simulink model "test_final_sift"  (R2015a)
settings: Solver=ode45  StartTime=0.0  StopTime=10.0  RelTol=1e-3
InitFcn:
  | %% DSPBuilder Start
  | alt_dspbuilder_update_model(bdroot)
  | %% DSPBuilder End
libraries: allblocks_alteradspbuilder2 x2309
(part 20 of 27)

== system test_final_sift/sift_octave1/get_descriptor/scale_space/Gaussian_scale4/line_buff ==
  dataIn : Inport
  clken : Inport  Port=2
  Delay : allblocks_alteradspbuilder2/Delay  pipeline=1  pipeline_display=1  ClockPhase=1  use_ena=on  use_sclr=off  allowFloatingPointOverride=on  logOutputs=off  logFile=C:\Users\ASUS\Desktop\sift_fpga\Octave_2\tb_test_final_sift\test%5Ffinal%5Fsift_sift%5Foctave1_get%5Fdescriptor_scale%5Fspace_Gaussian%5Fscale4_line%5Fbuff_Delay.fixedpointlog  use_init=off  reset_value=1
  Delay1 : allblocks_alteradspbuilder2/Delay  pipeline=1  pipeline_display=1  ClockPhase=1  use_ena=on  use_sclr=off  allowFloatingPointOverride=on  logOutputs=off  logFile=C:\Users\ASUS\Desktop\sift_fpga\Octave_2\tb_test_final_sift\test%5Ffinal%5Fsift_sift%5Foctave1_get%5Fdescriptor_scale%5Fspace_Gaussian%5Fscale4_line%5Fbuff_Delay1.fixedpointlog  use_init=off  reset_value=1
  Delay10 : allblocks_alteradspbuilder2/Delay  pipeline=1  pipeline_display=1  ClockPhase=1  use_ena=on  use_sclr=off  allowFloatingPointOverride=on  logOutputs=off  logFile=C:\Users\ASUS\Desktop\sift_fpga\Octave_2\tb_test_final_sift\test%5Ffinal%5Fsift_sift%5Foctave1_get%5Fdescriptor_scale%5Fspace_Gaussian%5Fscale4_line%5Fbuff_Delay10.fixedpointlog  use_init=off  reset_value=1
  Delay11 : allblocks_alteradspbuilder2/Delay  pipeline=1  pipeline_display=1  ClockPhase=1  use_ena=on  use_sclr=off  allowFloatingPointOverride=on  logOutputs=off  logFile=C:\Users\ASUS\Desktop\sift_fpga\Octave_2\tb_test_final_sift\test%5Ffinal%5Fsift_sift%5Foctave1_get%5Fdescriptor_scale%5Fspace_Gaussian%5Fscale4_line%5Fbuff_Delay11.fixedpointlog  use_init=off  reset_value=1
  Delay12 : allblocks_alteradspbuilder2/Delay  pipeline=1  pipeline_display=1  ClockPhase=1  use_ena=on  use_sclr=off  allowFloatingPointOverride=on  logOutputs=off  logFile=C:\Users\ASUS\Desktop\sift_fpga\Octave_2\tb_test_final_sift\test%5Ffinal%5Fsift_sift%5Foctave1_get%5Fdescriptor_scale%5Fspace_Gaussian%5Fscale4_line%5Fbuff_Delay12.fixedpointlog  use_init=off  reset_value=1
  Delay13 : allblocks_alteradspbuilder2/Delay  pipeline=1  pipeline_display=1  ClockPhase=1  use_ena=on  use_sclr=off  allowFloatingPointOverride=on  logOutputs=off  logFile=C:\Users\ASUS\Desktop\sift_fpga\Octave_2\tb_test_final_sift\test%5Ffinal%5Fsift_sift%5Foctave1_get%5Fdescriptor_scale%5Fspace_Gaussian%5Fscale4_line%5Fbuff_Delay13.fixedpointlog  use_init=off  reset_value=1
  Delay14 : allblocks_alteradspbuilder2/Delay  pipeline=1  pipeline_display=1  ClockPhase=1  use_ena=on  use_sclr=off  allowFloatingPointOverride=on  logOutputs=off  logFile=C:\Users\ASUS\Desktop\sift_fpga\Octave_2\tb_test_final_sift\test%5Ffinal%5Fsift_sift%5Foctave1_get%5Fdescriptor_scale%5Fspace_Gaussian%5Fscale4_line%5Fbuff_Delay14.fixedpointlog  use_init=off  reset_value=1
  Delay15 : allblocks_alteradspbuilder2/Delay  pipeline=1  pipeline_display=1  ClockPhase=1  use_ena=on  use_sclr=off  allowFloatingPointOverride=on  logOutputs=off  logFile=C:\Users\ASUS\Desktop\sift_fpga\Octave_2\tb_test_final_sift\test%5Ffinal%5Fsift_sift%5Foctave1_get%5Fdescriptor_scale%5Fspace_Gaussian%5Fscale4_line%5Fbuff_Delay15.fixedpointlog  use_init=off  reset_value=1
  Delay16 : allblocks_alteradspbuilder2/Delay  pipeline=1  pipeline_display=1  ClockPhase=1  use_ena=on  use_sclr=off  allowFloatingPointOverride=on  logOutputs=off  logFile=C:\Users\ASUS\Desktop\sift_fpga\Octave_2\tb_test_final_sift\test%5Ffinal%5Fsift_sift%5Foctave1_get%5Fdescriptor_scale%5Fspace_Gaussian%5Fscale4_line%5Fbuff_Delay16.fixedpointlog  use_init=off  reset_value=1
  Delay17 : allblocks_alteradspbuilder2/Delay  pipeline=1  pipeline_display=1  ClockPhase=1  use_ena=on  use_sclr=off  allowFloatingPointOverride=on  logOutputs=off  logFile=C:\Users\ASUS\Desktop\sift_fpga\Octave_2\tb_test_final_sift\test%5Ffinal%5Fsift_sift%5Foctave1_get%5Fdescriptor_scale%5Fspace_Gaussian%5Fscale4_line%5Fbuff_Delay17.fixedpointlog  use_init=off  reset_value=1
  Delay18 : allblocks_alteradspbuilder2/Delay  pipeline=1  pipeline_display=1  ClockPhase=1  use_ena=on  use_sclr=off  allowFloatingPointOverride=on  logOutputs=off  logFile=C:\Users\ASUS\Desktop\sift_fpga\Octave_2\tb_test_final_sift\test%5Ffinal%5Fsift_sift%5Foctave1_get%5Fdescriptor_scale%5Fspace_Gaussian%5Fscale4_line%5Fbuff_Delay18.fixedpointlog  use_init=off  reset_value=1
  Delay19 : allblocks_alteradspbuilder2/Delay  pipeline=1  pipeline_display=1  ClockPhase=1  use_ena=on  use_sclr=off  allowFloatingPointOverride=on  logOutputs=off  logFile=C:\Users\ASUS\Desktop\sift_fpga\Octave_2\tb_test_final_sift\test%5Ffinal%5Fsift_sift%5Foctave1_get%5Fdescriptor_scale%5Fspace_Gaussian%5Fscale4_line%5Fbuff_Delay19.fixedpointlog  use_init=off  reset_value=1
  Delay2 : allblocks_alteradspbuilder2/Delay  pipeline=1  pipeline_display=1  ClockPhase=1  use_ena=on  use_sclr=off  allowFloatingPointOverride=on  logOutputs=off  logFile=C:\Users\ASUS\Desktop\sift_fpga\Octave_2\tb_test_final_sift\test%5Ffinal%5Fsift_sift%5Foctave1_get%5Fdescriptor_scale%5Fspace_Gaussian%5Fscale4_line%5Fbuff_Delay2.fixedpointlog  use_init=off  reset_value=1
  Delay20 : allblocks_alteradspbuilder2/Delay  pipeline=1  pipeline_display=1  ClockPhase=1  use_ena=on  use_sclr=off  allowFloatingPointOverride=on  logOutputs=off  logFile=C:\Users\ASUS\Desktop\sift_fpga\Octave_2\tb_test_final_sift\test%5Ffinal%5Fsift_sift%5Foctave1_get%5Fdescriptor_scale%5Fspace_Gaussian%5Fscale4_line%5Fbuff_Delay20.fixedpointlog  use_init=off  reset_value=1
  Delay3 : allblocks_alteradspbuilder2/Delay  pipeline=1  pipeline_display=1  ClockPhase=1  use_ena=on  use_sclr=off  allowFloatingPointOverride=on  logOutputs=off  logFile=C:\Users\ASUS\Desktop\sift_fpga\Octave_2\tb_test_final_sift\test%5Ffinal%5Fsift_sift%5Foctave1_get%5Fdescriptor_scale%5Fspace_Gaussian%5Fscale4_line%5Fbuff_Delay3.fixedpointlog  use_init=off  reset_value=1
  Delay4 : allblocks_alteradspbuilder2/Delay  pipeline=1  pipeline_display=1  ClockPhase=1  use_ena=on  use_sclr=off  allowFloatingPointOverride=on  logOutputs=off  logFile=C:\Users\ASUS\Desktop\sift_fpga\Octave_2\tb_test_final_sift\test%5Ffinal%5Fsift_sift%5Foctave1_get%5Fdescriptor_scale%5Fspace_Gaussian%5Fscale4_line%5Fbuff_Delay4.fixedpointlog  use_init=off  reset_value=1
  Delay5 : allblocks_alteradspbuilder2/Delay  pipeline=1  pipeline_display=1  ClockPhase=1  use_ena=on  use_sclr=off  allowFloatingPointOverride=on  logOutputs=off  logFile=C:\Users\ASUS\Desktop\sift_fpga\Octave_2\tb_test_final_sift\test%5Ffinal%5Fsift_sift%5Foctave1_get%5Fdescriptor_scale%5Fspace_Gaussian%5Fscale4_line%5Fbuff_Delay5.fixedpointlog  use_init=off  reset_value=1
  Delay6 : allblocks_alteradspbuilder2/Delay  pipeline=1  pipeline_display=1  ClockPhase=1  use_ena=on  use_sclr=off  allowFloatingPointOverride=on  logOutputs=off  logFile=C:\Users\ASUS\Desktop\sift_fpga\Octave_2\tb_test_final_sift\test%5Ffinal%5Fsift_sift%5Foctave1_get%5Fdescriptor_scale%5Fspace_Gaussian%5Fscale4_line%5Fbuff_Delay6.fixedpointlog  use_init=off  reset_value=1
  Delay7 : allblocks_alteradspbuilder2/Delay  pipeline=1  pipeline_display=1  ClockPhase=1  use_ena=on  use_sclr=off  allowFloatingPointOverride=on  logOutputs=off  logFile=C:\Users\ASUS\Desktop\sift_fpga\Octave_2\tb_test_final_sift\test%5Ffinal%5Fsift_sift%5Foctave1_get%5Fdescriptor_scale%5Fspace_Gaussian%5Fscale4_line%5Fbuff_Delay7.fixedpointlog  use_init=off  reset_value=1
  Delay8 : allblocks_alteradspbuilder2/Delay  pipeline=1  pipeline_display=1  ClockPhase=1  use_ena=on  use_sclr=off  allowFloatingPointOverride=on  logOutputs=off  logFile=C:\Users\ASUS\Desktop\sift_fpga\Octave_2\tb_test_final_sift\test%5Ffinal%5Fsift_sift%5Foctave1_get%5Fdescriptor_scale%5Fspace_Gaussian%5Fscale4_line%5Fbuff_Delay8.fixedpointlog  use_init=off  reset_value=1
  Delay9 : allblocks_alteradspbuilder2/Delay  pipeline=1  pipeline_display=1  ClockPhase=1  use_ena=on  use_sclr=off  allowFloatingPointOverride=on  logOutputs=off  logFile=C:\Users\ASUS\Desktop\sift_fpga\Octave_2\tb_test_final_sift\test%5Ffinal%5Fsift_sift%5Foctave1_get%5Fdescriptor_scale%5Fspace_Gaussian%5Fscale4_line%5Fbuff_Delay9.fixedpointlog  use_init=off  reset_value=1
  Memory Delay : allblocks_alteradspbuilder2/Memory Delay  BusType=Unsigned Integer  bwl=8  bwr=0  pipeline=636  pipeline_display=636  ram_type=AUTO  use_ena=on  use_sclr=off  allowFloatingPointOverride=on  logOutputs=off  logFile=C:\Users\ASUS\Desktop\sift_fpga\Octave_2\tb_test_final_sift\test%5Ffinal%5Fsift_sift%5Foctave1_get%5Fdescriptor_scale%5Fspace_Gaussian%5Fscale4_line%5Fbuff_Memory+Delay.fixedpointlog
  Memory Delay1 : allblocks_alteradspbuilder2/Memory Delay  BusType=Unsigned Integer  bwl=8  bwr=0  pipeline=636  pipeline_display=636  ram_type=AUTO  use_ena=on  use_sclr=off  allowFloatingPointOverride=on  logOutputs=off  logFile=C:\Users\ASUS\Desktop\sift_fpga\Octave_2\tb_test_final_sift\test%5Ffinal%5Fsift_sift%5Foctave1_get%5Fdescriptor_scale%5Fspace_Gaussian%5Fscale4_line%5Fbuff_Memory+Delay1.fixedpointlog
  Memory Delay2 : allblocks_alteradspbuilder2/Memory Delay  BusType=Unsigned Integer  bwl=8  bwr=0  pipeline=636  pipeline_display=636  ram_type=AUTO  use_ena=on  use_sclr=off  allowFloatingPointOverride=on  logOutputs=off  logFile=C:\Users\ASUS\Desktop\sift_fpga\Octave_2\tb_test_final_sift\test%5Ffinal%5Fsift_sift%5Foctave1_get%5Fdescriptor_scale%5Fspace_Gaussian%5Fscale4_line%5Fbuff_Memory+Delay2.fixedpointlog
  Memory Delay3 : allblocks_alteradspbuilder2/Memory Delay  BusType=Unsigned Integer  bwl=8  bwr=0  pipeline=636  pipeline_display=636  ram_type=AUTO  use_ena=on  use_sclr=off  allowFloatingPointOverride=on  logOutputs=off  logFile=C:\Users\ASUS\Desktop\sift_fpga\Octave_2\tb_test_final_sift\test%5Ffinal%5Fsift_sift%5Foctave1_get%5Fdescriptor_scale%5Fspace_Gaussian%5Fscale4_line%5Fbuff_Memory+Delay3.fixedpointlog
  Out00 : Outport
  Out01 : Outport  Port=2
  Out02 : Outport  Port=3
  Out03 : Outport  Port=4
  Out04 : Outport  Port=5
  Out10 : Outport  Port=6
  Out11 : Outport  Port=7
  Out12 : Outport  Port=8
  Out13 : Outport  Port=9
  Out14 : Outport  Port=10
  Out20 : Outport  Port=11
  Out21 : Outport  Port=12
  Out22 : Outport  Port=13
  Out23 : Outport  Port=14
  Out24 : Outport  Port=15
  Out30 : Outport  Port=16
  Out31 : Outport  Port=17
  Out32 : Outport  Port=18
  Out33 : Outport  Port=19
  Out34 : Outport  Port=20
  Out40 : Outport  Port=21
  Out41 : Outport  Port=22
  Out42 : Outport  Port=23
  Out43 : Outport  Port=24
  Out44 : Outport  Port=25
  wires:
  [clken] -> Delay9/2
  [data_04] -> Out04/1
  [data_02] -> Out02/1
  [clken] -> Memory Delay1/2
  [data_44] -> Out44/1
  [data_33] -> Out33/1
  [clken] -> Delay4/2
  [clken] -> Delay11/2
  [data_32] -> Out32/1
  [data_31] -> Out31/1
  [data_40] -> Out40/1
  [data_43] -> Out43/1
  [data_42] -> Out42/1
  Delay11/1 -> [data_23], Delay12/1
  Memory Delay1/1 -> [data_20], Delay9/1
  [data_41] -> Out41/1
  Delay9/1 -> [data_21], Delay10/1
  [clken] -> Delay12/2
  [data_34] -> Out34/1
  [data_30] -> Out30/1
  Delay/1 -> [data_00], Delay1/1
  [clken] -> Delay1/2
  [clken] -> Delay/2
  [data_03] -> Out03/1
  [clken] -> Delay10/2
  Delay8/1 -> Memory Delay1/1, [data_14]
  Delay10/1 -> [data_22], Delay11/1
  [data_12] -> Out12/1
  dataIn/1 -> [data_in]
  Memory Delay3/1 -> [data_40], Delay20/1
  [clken] -> Memory Delay/2
  [clken] -> Delay2/2
  [data_22] -> Out22/1
  [clken] -> Delay14/2
  Delay17/1 -> [data_32], Delay18/1
  [clken] -> Delay20/2
  [data_10] -> Out10/1
  [data_21] -> Out21/1
  Delay12/1 -> [data_24], Memory Delay2/1
  Delay4/1 -> Memory Delay/1, [data_04]
  [clken] -> Delay3/2
  Delay2/1 -> [data_02], Delay3/1
  [clken] -> Memory Delay2/2
  [data_23] -> Out23/1
  [data_13] -> Out13/1
  clken/1 -> [clken]
  [data_11] -> Out11/1
  Delay18/1 -> [data_33], Delay19/1
  [data_20] -> Out20/1
  Delay1/1 -> [data_01], Delay2/1
  [data_24] -> Out24/1
  Memory Delay2/1 -> [data_30], Delay16/1
  [clken] -> Delay16/2
  [data_14] -> Out14/1
  [data_00] -> Out00/1
  [clken] -> Delay15/2
  [clken] -> Memory Delay3/2
  [data_01] -> Out01/1
  [data_in] -> Delay/1
  [clken] -> Delay7/2
  Delay19/1 -> Memory Delay3/1, [data_34]
  Delay14/1 -> [data_43], Delay15/1
  Memory Delay/1 -> [data_10], Delay5/1
  Delay5/1 -> [data_11], Delay6/1
  Delay16/1 -> [data_31], Delay17/1
  [clken] -> Delay6/2
  Delay6/1 -> [data_12], Delay7/1
  [clken] -> Delay13/2
  Delay3/1 -> [data_03], Delay4/1
  Delay15/1 -> [data_44]
  [clken] -> Delay18/2
  Delay13/1 -> [data_42], Delay14/1
  [clken] -> Delay5/2
  Delay7/1 -> [data_13], Delay8/1
  Delay20/1 -> [data_41], Delay13/1
  [clken] -> Delay17/2
  [clken] -> Delay19/2
  [clken] -> Delay8/2

== system test_final_sift/sift_octave1/matching/compare_descriptor/get_distance/BusSplitter ==
  data_in : Inport
  AltBus : allblocks_alteradspbuilder2/AltBus  BusType=Unsigned Integer  bwl=112  bwr=0  saturate=off  floatingPointInput=on  floatingPointOutput=on  logOutputs=off  logFile=C:\Users\ASUS\Desktop\sift_fpga\Octave_2\tb_test_final_sift\test%5Ffinal%5Fsift_sift%5Foctave1_matching_compare%5Fdescriptor_get%5Fdistance_BusSplitter_AltBus.fixedpointlog
  AltBus1 : allblocks_alteradspbuilder2/AltBus  BusType=Unsigned Integer  bwl=96  bwr=0  saturate=off  floatingPointInput=on  floatingPointOutput=on  logOutputs=off  logFile=C:\Users\ASUS\Desktop\sift_fpga\Octave_2\tb_test_final_sift\test%5Ffinal%5Fsift_sift%5Foctave1_matching_compare%5Fdescriptor_get%5Fdistance_BusSplitter_AltBus1.fixedpointlog
  AltBus10 : allblocks_alteradspbuilder2/AltBus  BusType=Unsigned Integer  bwl=16  bwr=0  saturate=off  floatingPointInput=on  floatingPointOutput=on  logOutputs=off  logFile=C:\Users\ASUS\Desktop\sift_fpga\Octave_2\tb_test_final_sift\test%5Ffinal%5Fsift_sift%5Foctave1_matching_compare%5Fdescriptor_get%5Fdistance_BusSplitter_AltBus10.fixedpointlog
  AltBus11 : allblocks_alteradspbuilder2/AltBus  BusType=Unsigned Integer  bwl=16  bwr=0  saturate=off  floatingPointInput=on  floatingPointOutput=on  logOutputs=off  logFile=C:\Users\ASUS\Desktop\sift_fpga\Octave_2\tb_test_final_sift\test%5Ffinal%5Fsift_sift%5Foctave1_matching_compare%5Fdescriptor_get%5Fdistance_BusSplitter_AltBus11.fixedpointlog
  AltBus12 : allblocks_alteradspbuilder2/AltBus  BusType=Unsigned Integer  bwl=16  bwr=0  saturate=off  floatingPointInput=on  floatingPointOutput=on  logOutputs=off  logFile=C:\Users\ASUS\Desktop\sift_fpga\Octave_2\tb_test_final_sift\test%5Ffinal%5Fsift_sift%5Foctave1_matching_compare%5Fdescriptor_get%5Fdistance_BusSplitter_AltBus12.fixedpointlog
  AltBus13 : allblocks_alteradspbuilder2/AltBus  BusType=Unsigned Integer  bwl=16  bwr=0  saturate=off  floatingPointInput=on  floatingPointOutput=on  logOutputs=off  logFile=C:\Users\ASUS\Desktop\sift_fpga\Octave_2\tb_test_final_sift\test%5Ffinal%5Fsift_sift%5Foctave1_matching_compare%5Fdescriptor_get%5Fdistance_BusSplitter_AltBus13.fixedpointlog
  AltBus2 : allblocks_alteradspbuilder2/AltBus  BusType=Unsigned Integer  bwl=80  bwr=0  saturate=off  floatingPointInput=on  floatingPointOutput=on  logOutputs=off  logFile=C:\Users\ASUS\Desktop\sift_fpga\Octave_2\tb_test_final_sift\test%5Ffinal%5Fsift_sift%5Foctave1_matching_compare%5Fdescriptor_get%5Fdistance_BusSplitter_AltBus2.fixedpointlog
  AltBus3 : allblocks_alteradspbuilder2/AltBus  BusType=Unsigned Integer  bwl=64  bwr=0  saturate=off  floatingPointInput=on  floatingPointOutput=on  logOutputs=off  logFile=C:\Users\ASUS\Desktop\sift_fpga\Octave_2\tb_test_final_sift\test%5Ffinal%5Fsift_sift%5Foctave1_matching_compare%5Fdescriptor_get%5Fdistance_BusSplitter_AltBus3.fixedpointlog
  AltBus4 : allblocks_alteradspbuilder2/AltBus  BusType=Unsigned Integer  bwl=48  bwr=0  saturate=off  floatingPointInput=on  floatingPointOutput=on  logOutputs=off  logFile=C:\Users\ASUS\Desktop\sift_fpga\Octave_2\tb_test_final_sift\test%5Ffinal%5Fsift_sift%5Foctave1_matching_compare%5Fdescriptor_get%5Fdistance_BusSplitter_AltBus4.fixedpointlog
  AltBus5 : allblocks_alteradspbuilder2/AltBus  BusType=Unsigned Integer  bwl=32  bwr=0  saturate=off  floatingPointInput=on  floatingPointOutput=on  logOutputs=off  logFile=C:\Users\ASUS\Desktop\sift_fpga\Octave_2\tb_test_final_sift\test%5Ffinal%5Fsift_sift%5Foctave1_matching_compare%5Fdescriptor_get%5Fdistance_BusSplitter_AltBus5.fixedpointlog
  AltBus6 : allblocks_alteradspbuilder2/AltBus  BusType=Unsigned Integer  bwl=16  bwr=0  saturate=off  floatingPointInput=on  floatingPointOutput=on  logOutputs=off  logFile=C:\Users\ASUS\Desktop\sift_fpga\Octave_2\tb_test_final_sift\test%5Ffinal%5Fsift_sift%5Foctave1_matching_compare%5Fdescriptor_get%5Fdistance_BusSplitter_AltBus6.fixedpointlog
  AltBus7 : allblocks_alteradspbuilder2/AltBus  BusType=Unsigned Integer  bwl=16  bwr=0  saturate=off  floatingPointInput=on  floatingPointOutput=on  logOutputs=off  logFile=C:\Users\ASUS\Desktop\sift_fpga\Octave_2\tb_test_final_sift\test%5Ffinal%5Fsift_sift%5Foctave1_matching_compare%5Fdescriptor_get%5Fdistance_BusSplitter_AltBus7.fixedpointlog
  AltBus8 : allblocks_alteradspbuilder2/AltBus  BusType=Unsigned Integer  bwl=16  bwr=0  saturate=off  floatingPointInput=on  floatingPointOutput=on  logOutputs=off  logFile=C:\Users\ASUS\Desktop\sift_fpga\Octave_2\tb_test_final_sift\test%5Ffinal%5Fsift_sift%5Foctave1_matching_compare%5Fdescriptor_get%5Fdistance_BusSplitter_AltBus8.fixedpointlog
  AltBus9 : allblocks_alteradspbuilder2/AltBus  BusType=Unsigned Integer  bwl=16  bwr=0  saturate=off  floatingPointInput=on  floatingPointOutput=on  logOutputs=off  logFile=C:\Users\ASUS\Desktop\sift_fpga\Octave_2\tb_test_final_sift\test%5Ffinal%5Fsift_sift%5Foctave1_matching_compare%5Fdescriptor_get%5Fdistance_BusSplitter_AltBus9.fixedpointlog
  Logical Bus Operator : allblocks_alteradspbuilder2/Logical Bus Operator  BusType=Unsigned Integer  bwl=128  bwr=0  LogicalOp_text=Shift Right  mask_value_num=-5  shift_amount=112  force_sign_ext=off  pipeline_display=0
  Logical Bus Operator1 : allblocks_alteradspbuilder2/Logical Bus Operator  BusType=Unsigned Integer  bwl=112  bwr=0  LogicalOp_text=Shift Right  mask_value_num=-5  shift_amount=96  force_sign_ext=off  pipeline_display=0
  Logical Bus Operator2 : allblocks_alteradspbuilder2/Logical Bus Operator  BusType=Unsigned Integer  bwl=96  bwr=0  LogicalOp_text=Shift Right  mask_value_num=-5  shift_amount=80  force_sign_ext=off  pipeline_display=0
  Logical Bus Operator3 : allblocks_alteradspbuilder2/Logical Bus Operator  BusType=Unsigned Integer  bwl=80  bwr=0  LogicalOp_text=Shift Right  mask_value_num=-5  shift_amount=64  force_sign_ext=off  pipeline_display=0
  Logical Bus Operator4 : allblocks_alteradspbuilder2/Logical Bus Operator  BusType=Unsigned Integer  bwl=64  bwr=0  LogicalOp_text=Shift Right  mask_value_num=-5  shift_amount=48  force_sign_ext=off  pipeline_display=0
  Logical Bus Operator5 : allblocks_alteradspbuilder2/Logical Bus Operator  BusType=Unsigned Integer  bwl=48  bwr=0  LogicalOp_text=Shift Right  mask_value_num=-5  shift_amount=32  force_sign_ext=off  pipeline_display=0
  Logical Bus Operator6 : allblocks_alteradspbuilder2/Logical Bus Operator  BusType=Unsigned Integer  bwl=32  bwr=0  LogicalOp_text=Shift Right  mask_value_num=-5  shift_amount=16  force_sign_ext=off  pipeline_display=0
  bin1 : Outport
  bin2 : Outport  Port=2
  bin3 : Outport  Port=3
  bin4 : Outport  Port=4
  bin5 : Outport  Port=5
  bin6 : Outport  Port=6
  bin7 : Outport  Port=7
  bin8 : Outport  Port=8
  wires:
  Logical Bus Operator6/1 -> AltBus7/1
  AltBus1/1 -> Logical Bus Operator2/1
  AltBus9/1 -> bin5/1
  AltBus8/1 -> bin6/1
  AltBus7/1 -> bin7/1
  AltBus6/1 -> bin8/1
  AltBus/1 -> Logical Bus Operator1/1
  AltBus10/1 -> bin4/1
  AltBus12/1 -> bin3/1
  AltBus11/1 -> bin1/1
  AltBus3/1 -> Logical Bus Operator4/1
  AltBus2/1 -> Logical Bus Operator3/1
  AltBus4/1 -> Logical Bus Operator5/1
  data_in/1 -> AltBus6/1, AltBus5/1, AltBus4/1, AltBus3/1, AltBus2/1, AltBus1/1, AltBus/1, Logical Bus Operator/1
  AltBus5/1 -> Logical Bus Operator6/1
  Logical Bus Operator1/1 -> AltBus13/1
  Logical Bus Operator2/1 -> AltBus12/1
  Logical Bus Operator/1 -> AltBus11/1
  Logical Bus Operator5/1 -> AltBus8/1
  Logical Bus Operator4/1 -> AltBus9/1
  Logical Bus Operator3/1 -> AltBus10/1
  AltBus13/1 -> bin2/1

== system test_final_sift/sift_octave1/matching/compare_descriptor/get_distance/BusSplitter1 ==
  data_in : Inport
  AltBus : allblocks_alteradspbuilder2/AltBus  BusType=Unsigned Integer  bwl=112  bwr=0  saturate=off  floatingPointInput=on  floatingPointOutput=on  logOutputs=off  logFile=C:\Users\ASUS\Desktop\sift_fpga\Octave_2\tb_test_final_sift\test%5Ffinal%5Fsift_sift%5Foctave1_matching_compare%5Fdescriptor_get%5Fdistance_BusSplitter1_AltBus.fixedpointlog
  AltBus1 : allblocks_alteradspbuilder2/AltBus  BusType=Unsigned Integer  bwl=96  bwr=0  saturate=off  floatingPointInput=on  floatingPointOutput=on  logOutputs=off  logFile=C:\Users\ASUS\Desktop\sift_fpga\Octave_2\tb_test_final_sift\test%5Ffinal%5Fsift_sift%5Foctave1_matching_compare%5Fdescriptor_get%5Fdistance_BusSplitter1_AltBus1.fixedpointlog
  AltBus10 : allblocks_alteradspbuilder2/AltBus  BusType=Unsigned Integer  bwl=16  bwr=0  saturate=off  floatingPointInput=on  floatingPointOutput=on  logOutputs=off  logFile=C:\Users\ASUS\Desktop\sift_fpga\Octave_2\tb_test_final_sift\test%5Ffinal%5Fsift_sift%5Foctave1_matching_compare%5Fdescriptor_get%5Fdistance_BusSplitter1_AltBus10.fixedpointlog
  AltBus11 : allblocks_alteradspbuilder2/AltBus  BusType=Unsigned Integer  bwl=16  bwr=0  saturate=off  floatingPointInput=on  floatingPointOutput=on  logOutputs=off  logFile=C:\Users\ASUS\Desktop\sift_fpga\Octave_2\tb_test_final_sift\test%5Ffinal%5Fsift_sift%5Foctave1_matching_compare%5Fdescriptor_get%5Fdistance_BusSplitter1_AltBus11.fixedpointlog
  AltBus12 : allblocks_alteradspbuilder2/AltBus  BusType=Unsigned Integer  bwl=16  bwr=0  saturate=off  floatingPointInput=on  floatingPointOutput=on  logOutputs=off  logFile=C:\Users\ASUS\Desktop\sift_fpga\Octave_2\tb_test_final_sift\test%5Ffinal%5Fsift_sift%5Foctave1_matching_compare%5Fdescriptor_get%5Fdistance_BusSplitter1_AltBus12.fixedpointlog
  AltBus13 : allblocks_alteradspbuilder2/AltBus  BusType=Unsigned Integer  bwl=16  bwr=0  saturate=off  floatingPointInput=on  floatingPointOutput=on  logOutputs=off  logFile=C:\Users\ASUS\Desktop\sift_fpga\Octave_2\tb_test_final_sift\test%5Ffinal%5Fsift_sift%5Foctave1_matching_compare%5Fdescriptor_get%5Fdistance_BusSplitter1_AltBus13.fixedpointlog
  AltBus2 : allblocks_alteradspbuilder2/AltBus  BusType=Unsigned Integer  bwl=80  bwr=0  saturate=off  floatingPointInput=on  floatingPointOutput=on  logOutputs=off  logFile=C:\Users\ASUS\Desktop\sift_fpga\Octave_2\tb_test_final_sift\test%5Ffinal%5Fsift_sift%5Foctave1_matching_compare%5Fdescriptor_get%5Fdistance_BusSplitter1_AltBus2.fixedpointlog
  AltBus3 : allblocks_alteradspbuilder2/AltBus  BusType=Unsigned Integer  bwl=64  bwr=0  saturate=off  floatingPointInput=on  floatingPointOutput=on  logOutputs=off  logFile=C:\Users\ASUS\Desktop\sift_fpga\Octave_2\tb_test_final_sift\test%5Ffinal%5Fsift_sift%5Foctave1_matching_compare%5Fdescriptor_get%5Fdistance_BusSplitter1_AltBus3.fixedpointlog
  AltBus4 : allblocks_alteradspbuilder2/AltBus  BusType=Unsigned Integer  bwl=48  bwr=0  saturate=off  floatingPointInput=on  floatingPointOutput=on  logOutputs=off  logFile=C:\Users\ASUS\Desktop\sift_fpga\Octave_2\tb_test_final_sift\test%5Ffinal%5Fsift_sift%5Foctave1_matching_compare%5Fdescriptor_get%5Fdistance_BusSplitter1_AltBus4.fixedpointlog
  AltBus5 : allblocks_alteradspbuilder2/AltBus  BusType=Unsigned Integer  bwl=32  bwr=0  saturate=off  floatingPointInput=on  floatingPointOutput=on  logOutputs=off  logFile=C:\Users\ASUS\Desktop\sift_fpga\Octave_2\tb_test_final_sift\test%5Ffinal%5Fsift_sift%5Foctave1_matching_compare%5Fdescriptor_get%5Fdistance_BusSplitter1_AltBus5.fixedpointlog
  AltBus6 : allblocks_alteradspbuilder2/AltBus  BusType=Unsigned Integer  bwl=16  bwr=0  saturate=off  floatingPointInput=on  floatingPointOutput=on  logOutputs=off  logFile=C:\Users\ASUS\Desktop\sift_fpga\Octave_2\tb_test_final_sift\test%5Ffinal%5Fsift_sift%5Foctave1_matching_compare%5Fdescriptor_get%5Fdistance_BusSplitter1_AltBus6.fixedpointlog
  AltBus7 : allblocks_alteradspbuilder2/AltBus  BusType=Unsigned Integer  bwl=16  bwr=0  saturate=off  floatingPointInput=on  floatingPointOutput=on  logOutputs=off  logFile=C:\Users\ASUS\Desktop\sift_fpga\Octave_2\tb_test_final_sift\test%5Ffinal%5Fsift_sift%5Foctave1_matching_compare%5Fdescriptor_get%5Fdistance_BusSplitter1_AltBus7.fixedpointlog
  AltBus8 : allblocks_alteradspbuilder2/AltBus  BusType=Unsigned Integer  bwl=16  bwr=0  saturate=off  floatingPointInput=on  floatingPointOutput=on  logOutputs=off  logFile=C:\Users\ASUS\Desktop\sift_fpga\Octave_2\tb_test_final_sift\test%5Ffinal%5Fsift_sift%5Foctave1_matching_compare%5Fdescriptor_get%5Fdistance_BusSplitter1_AltBus8.fixedpointlog
  AltBus9 : allblocks_alteradspbuilder2/AltBus  BusType=Unsigned Integer  bwl=16  bwr=0  saturate=off  floatingPointInput=on  floatingPointOutput=on  logOutputs=off  logFile=C:\Users\ASUS\Desktop\sift_fpga\Octave_2\tb_test_final_sift\test%5Ffinal%5Fsift_sift%5Foctave1_matching_compare%5Fdescriptor_get%5Fdistance_BusSplitter1_AltBus9.fixedpointlog
  Logical Bus Operator : allblocks_alteradspbuilder2/Logical Bus Operator  BusType=Unsigned Integer  bwl=128  bwr=0  LogicalOp_text=Shift Right  mask_value_num=-5  shift_amount=112  force_sign_ext=off  pipeline_display=0
  Logical Bus Operator1 : allblocks_alteradspbuilder2/Logical Bus Operator  BusType=Unsigned Integer  bwl=112  bwr=0  LogicalOp_text=Shift Right  mask_value_num=-5  shift_amount=96  force_sign_ext=off  pipeline_display=0
  Logical Bus Operator2 : allblocks_alteradspbuilder2/Logical Bus Operator  BusType=Unsigned Integer  bwl=96  bwr=0  LogicalOp_text=Shift Right  mask_value_num=-5  shift_amount=80  force_sign_ext=off  pipeline_display=0
  Logical Bus Operator3 : allblocks_alteradspbuilder2/Logical Bus Operator  BusType=Unsigned Integer  bwl=80  bwr=0  LogicalOp_text=Shift Right  mask_value_num=-5  shift_amount=64  force_sign_ext=off  pipeline_display=0
  Logical Bus Operator4 : allblocks_alteradspbuilder2/Logical Bus Operator  BusType=Unsigned Integer  bwl=64  bwr=0  LogicalOp_text=Shift Right  mask_value_num=-5  shift_amount=48  force_sign_ext=off  pipeline_display=0
  Logical Bus Operator5 : allblocks_alteradspbuilder2/Logical Bus Operator  BusType=Unsigned Integer  bwl=48  bwr=0  LogicalOp_text=Shift Right  mask_value_num=-5  shift_amount=32  force_sign_ext=off  pipeline_display=0
  Logical Bus Operator6 : allblocks_alteradspbuilder2/Logical Bus Operator  BusType=Unsigned Integer  bwl=32  bwr=0  LogicalOp_text=Shift Right  mask_value_num=-5  shift_amount=16  force_sign_ext=off  pipeline_display=0
  bin1 : Outport
  bin2 : Outport  Port=2
  bin3 : Outport  Port=3
  bin4 : Outport  Port=4
  bin5 : Outport  Port=5
  bin6 : Outport  Port=6
  bin7 : Outport  Port=7
  bin8 : Outport  Port=8
  wires:
  Logical Bus Operator6/1 -> AltBus7/1
  AltBus1/1 -> Logical Bus Operator2/1
  AltBus9/1 -> bin5/1
  AltBus8/1 -> bin6/1
  AltBus7/1 -> bin7/1
  AltBus6/1 -> bin8/1
  AltBus/1 -> Logical Bus Operator1/1
  AltBus10/1 -> bin4/1
  AltBus12/1 -> bin3/1
  AltBus11/1 -> bin1/1
  AltBus3/1 -> Logical Bus Operator4/1
  AltBus2/1 -> Logical Bus Operator3/1
  AltBus4/1 -> Logical Bus Operator5/1
  data_in/1 -> AltBus6/1, AltBus5/1, AltBus4/1, AltBus3/1, AltBus2/1, AltBus1/1, AltBus/1, Logical Bus Operator/1
  AltBus5/1 -> Logical Bus Operator6/1
  Logical Bus Operator1/1 -> AltBus13/1
  Logical Bus Operator2/1 -> AltBus12/1
  Logical Bus Operator/1 -> AltBus11/1
  Logical Bus Operator5/1 -> AltBus8/1
  Logical Bus Operator4/1 -> AltBus9/1
  Logical Bus Operator3/1 -> AltBus10/1
  AltBus13/1 -> bin2/1

== system test_final_sift/sift_octave1/matching/compare_descriptor/get_distance/sub_GradOrian ==
  bin1 : Inport
  bin2 : Inport  Port=2
  clken : Inport  Port=3
  Comparator3 : allblocks_alteradspbuilder2/Comparator  direction=a > b  pipeline_display=0  allowFloatingPointOverride=on  logOutputs=off  logFile=C:\Users\ASUS\Desktop\sift_fpga\Octave_2\tb_test_final_sift\test%5Ffinal%5Fsift_sift%5Foctave1_matching_compare%5Fdescriptor_get%5Fdistance_sub%5FGradOrian_Comparator3.fixedpointlog
  Delay : allblocks_alteradspbuilder2/Delay  pipeline=1  pipeline_display=1  ClockPhase=1  use_ena=on  use_sclr=off  allowFloatingPointOverride=on  logOutputs=off  logFile=C:\Users\ASUS\Desktop\sift_fpga\Octave_2\tb_test_final_sift\test%5Ffinal%5Fsift_sift%5Foctave1_matching_compare%5Fdescriptor_get%5Fdistance_sub%5FGradOrian_Delay.fixedpointlog  use_init=off  reset_value=1
  Multiplexer2 : allblocks_alteradspbuilder2/Multiplexer  numInputs=2  pipeline=0  oneHot=off  pipeline_display=0  use_ena=off  use_aclr=off  allowFloatingPointOverride=on  logOutputs=off  logFile=C:\Users\ASUS\Desktop\sift_fpga\Octave_2\tb_test_final_sift\test%5Ffinal%5Fsift_sift%5Foctave1_matching_compare%5Fdescriptor_get%5Fdistance_sub%5FGradOrian_Multiplexer2.fixedpointlog
  Parallel Adder Subtractor : allblocks_alteradspbuilder2/Parallel Adder Subtractor  number_of_inputs=2  direction=+-  use_pipeline=on  pipeline_display=1  phase_selection=1  use_ena=on  use_aclr=off  allowFloatingPointOverride=on  logOutputs=off  logFile=C:\Users\ASUS\Desktop\sift_fpga\Octave_2\tb_test_final_sift\test%5Ffinal%5Fsift_sift%5Foctave1_matching_compare%5Fdescriptor_get%5Fdistance_sub%5FGradOrian_Parallel+Adder+Subtractor.fixedpointlog
  Parallel Adder Subtractor1 : allblocks_alteradspbuilder2/Parallel Adder Subtractor  number_of_inputs=2  direction=+-  use_pipeline=on  pipeline_display=1  phase_selection=1  use_ena=on  use_aclr=off  allowFloatingPointOverride=on  logOutputs=off  logFile=C:\Users\ASUS\Desktop\sift_fpga\Octave_2\tb_test_final_sift\test%5Ffinal%5Fsift_sift%5Foctave1_matching_compare%5Fdescriptor_get%5Fdistance_sub%5FGradOrian_Parallel+Adder+Subtractor1.fixedpointlog
  sub_bin : Outport
  wires:
  Comparator3/1 -> Delay/1
  [bin2] -> Comparator3/2
  [bin1] -> Comparator3/1
  Delay/1 -> Multiplexer2/1
  [clken] -> Delay/2
  [bin2] -> Parallel Adder Subtractor/2
  [bin1] -> Parallel Adder Subtractor1/2
  [bin2] -> Parallel Adder Subtractor1/1
  [clken] -> Parallel Adder Subtractor/3
  Parallel Adder Subtractor/1 -> [bin12]
  Parallel Adder Subtractor1/1 -> [bin21]
  [clken] -> Parallel Adder Subtractor1/3
  [bin1] -> Parallel Adder Subtractor/1
  bin1/1 -> [bin1]
  bin2/1 -> [bin2]
  [bin12] -> Multiplexer2/3
  [bin21] -> Multiplexer2/2
  Multiplexer2/1 -> sub_bin/1
  clken/1 -> [clken]

== system test_final_sift/sift_octave1/matching/compare_descriptor/get_distance/sub_GradOrian1 ==
  bin1 : Inport
  bin2 : Inport  Port=2
  clken : Inport  Port=3
  Comparator3 : allblocks_alteradspbuilder2/Comparator  direction=a > b  pipeline_display=0  allowFloatingPointOverride=on  logOutputs=off  logFile=C:\Users\ASUS\Desktop\sift_fpga\Octave_2\tb_test_final_sift\test%5Ffinal%5Fsift_sift%5Foctave1_matching_compare%5Fdescriptor_get%5Fdistance_sub%5FGradOrian1_Comparator3.fixedpointlog
  Delay : allblocks_alteradspbuilder2/Delay  pipeline=1  pipeline_display=1  ClockPhase=1  use_ena=on  use_sclr=off  allowFloatingPointOverride=on  logOutputs=off  logFile=C:\Users\ASUS\Desktop\sift_fpga\Octave_2\tb_test_final_sift\test%5Ffinal%5Fsift_sift%5Foctave1_matching_compare%5Fdescriptor_get%5Fdistance_sub%5FGradOrian1_Delay.fixedpointlog  use_init=off  reset_value=1
  Multiplexer2 : allblocks_alteradspbuilder2/Multiplexer  numInputs=2  pipeline=0  oneHot=off  pipeline_display=0  use_ena=off  use_aclr=off  allowFloatingPointOverride=on  logOutputs=off  logFile=C:\Users\ASUS\Desktop\sift_fpga\Octave_2\tb_test_final_sift\test%5Ffinal%5Fsift_sift%5Foctave1_matching_compare%5Fdescriptor_get%5Fdistance_sub%5FGradOrian1_Multiplexer2.fixedpointlog
  Parallel Adder Subtractor : allblocks_alteradspbuilder2/Parallel Adder Subtractor  number_of_inputs=2  direction=+-  use_pipeline=on  pipeline_display=1  phase_selection=1  use_ena=on  use_aclr=off  allowFloatingPointOverride=on  logOutputs=off  logFile=C:\Users\ASUS\Desktop\sift_fpga\Octave_2\tb_test_final_sift\test%5Ffinal%5Fsift_sift%5Foctave1_matching_compare%5Fdescriptor_get%5Fdistance_sub%5FGradOrian1_Parallel+Adder+Subtractor.fixedpointlog
  Parallel Adder Subtractor1 : allblocks_alteradspbuilder2/Parallel Adder Subtractor  number_of_inputs=2  direction=+-  use_pipeline=on  pipeline_display=1  phase_selection=1  use_ena=on  use_aclr=off  allowFloatingPointOverride=on  logOutputs=off  logFile=C:\Users\ASUS\Desktop\sift_fpga\Octave_2\tb_test_final_sift\test%5Ffinal%5Fsift_sift%5Foctave1_matching_compare%5Fdescriptor_get%5Fdistance_sub%5FGradOrian1_Parallel+Adder+Subtractor1.fixedpointlog
  sub_bin : Outport
  wires:
  Comparator3/1 -> Delay/1
  [bin2] -> Comparator3/2
  [bin1] -> Comparator3/1
  Delay/1 -> Multiplexer2/1
  [clken] -> Delay/2
  [bin2] -> Parallel Adder Subtractor/2
  [bin1] -> Parallel Adder Subtractor1/2
  [bin2] -> Parallel Adder Subtractor1/1
  [clken] -> Parallel Adder Subtractor/3
  Parallel Adder Subtractor/1 -> [bin12]
  Parallel Adder Subtractor1/1 -> [bin21]
  [clken] -> Parallel Adder Subtractor1/3
  [bin1] -> Parallel Adder Subtractor/1
  bin1/1 -> [bin1]
  bin2/1 -> [bin2]
  [bin12] -> Multiplexer2/3
  [bin21] -> Multiplexer2/2
  Multiplexer2/1 -> sub_bin/1
  clken/1 -> [clken]

== system test_final_sift/sift_octave1/matching/compare_descriptor/get_distance/sub_GradOrian2 ==
  bin1 : Inport
  bin2 : Inport  Port=2
  clken : Inport  Port=3
  Comparator3 : allblocks_alteradspbuilder2/Comparator  direction=a > b  pipeline_display=0  allowFloatingPointOverride=on  logOutputs=off  logFile=C:\Users\ASUS\Desktop\sift_fpga\Octave_2\tb_test_final_sift\test%5Ffinal%5Fsift_sift%5Foctave1_matching_compare%5Fdescriptor_get%5Fdistance_sub%5FGradOrian2_Comparator3.fixedpointlog
  Delay : allblocks_alteradspbuilder2/Delay  pipeline=1  pipeline_display=1  ClockPhase=1  use_ena=on  use_sclr=off  allowFloatingPointOverride=on  logOutputs=off  logFile=C:\Users\ASUS\Desktop\sift_fpga\Octave_2\tb_test_final_sift\test%5Ffinal%5Fsift_sift%5Foctave1_matching_compare%5Fdescriptor_get%5Fdistance_sub%5FGradOrian2_Delay.fixedpointlog  use_init=off  reset_value=1
  Multiplexer2 : allblocks_alteradspbuilder2/Multiplexer  numInputs=2  pipeline=0  oneHot=off  pipeline_display=0  use_ena=off  use_aclr=off  allowFloatingPointOverride=on  logOutputs=off  logFile=C:\Users\ASUS\Desktop\sift_fpga\Octave_2\tb_test_final_sift\test%5Ffinal%5Fsift_sift%5Foctave1_matching_compare%5Fdescriptor_get%5Fdistance_sub%5FGradOrian2_Multiplexer2.fixedpointlog
  Parallel Adder Subtractor : allblocks_alteradspbuilder2/Parallel Adder Subtractor  number_of_inputs=2  direction=+-  use_pipeline=on  pipeline_display=1  phase_selection=1  use_ena=on  use_aclr=off  allowFloatingPointOverride=on  logOutputs=off  logFile=C:\Users\ASUS\Desktop\sift_fpga\Octave_2\tb_test_final_sift\test%5Ffinal%5Fsift_sift%5Foctave1_matching_compare%5Fdescriptor_get%5Fdistance_sub%5FGradOrian2_Parallel+Adder+Subtractor.fixedpointlog
  Parallel Adder Subtractor1 : allblocks_alteradspbuilder2/Parallel Adder Subtractor  number_of_inputs=2  direction=+-  use_pipeline=on  pipeline_display=1  phase_selection=1  use_ena=on  use_aclr=off  allowFloatingPointOverride=on  logOutputs=off  logFile=C:\Users\ASUS\Desktop\sift_fpga\Octave_2\tb_test_final_sift\test%5Ffinal%5Fsift_sift%5Foctave1_matching_compare%5Fdescriptor_get%5Fdistance_sub%5FGradOrian2_Parallel+Adder+Subtractor1.fixedpointlog
  sub_bin : Outport
  wires:
  Comparator3/1 -> Delay/1
  [bin2] -> Comparator3/2
  [bin1] -> Comparator3/1
  Delay/1 -> Multiplexer2/1
  [clken] -> Delay/2
  [bin2] -> Parallel Adder Subtractor/2
  [bin1] -> Parallel Adder Subtractor1/2
  [bin2] -> Parallel Adder Subtractor1/1
  [clken] -> Parallel Adder Subtractor/3
  Parallel Adder Subtractor/1 -> [bin12]
  Parallel Adder Subtractor1/1 -> [bin21]
  [clken] -> Parallel Adder Subtractor1/3
  [bin1] -> Parallel Adder Subtractor/1
  bin1/1 -> [bin1]
  bin2/1 -> [bin2]
  [bin12] -> Multiplexer2/3
  [bin21] -> Multiplexer2/2
  Multiplexer2/1 -> sub_bin/1
  clken/1 -> [clken]

== system test_final_sift/sift_octave1/matching/compare_descriptor/get_distance/sub_GradOrian3 ==
  bin1 : Inport
  bin2 : Inport  Port=2
  clken : Inport  Port=3
  Comparator3 : allblocks_alteradspbuilder2/Comparator  direction=a > b  pipeline_display=0  allowFloatingPointOverride=on  logOutputs=off  logFile=C:\Users\ASUS\Desktop\sift_fpga\Octave_2\tb_test_final_sift\test%5Ffinal%5Fsift_sift%5Foctave1_matching_compare%5Fdescriptor_get%5Fdistance_sub%5FGradOrian3_Comparator3.fixedpointlog
  Delay : allblocks_alteradspbuilder2/Delay  pipeline=1  pipeline_display=1  ClockPhase=1  use_ena=on  use_sclr=off  allowFloatingPointOverride=on  logOutputs=off  logFile=C:\Users\ASUS\Desktop\sift_fpga\Octave_2\tb_test_final_sift\test%5Ffinal%5Fsift_sift%5Foctave1_matching_compare%5Fdescriptor_get%5Fdistance_sub%5FGradOrian3_Delay.fixedpointlog  use_init=off  reset_value=1
  Multiplexer2 : allblocks_alteradspbuilder2/Multiplexer  numInputs=2  pipeline=0  oneHot=off  pipeline_display=0  use_ena=off  use_aclr=off  allowFloatingPointOverride=on  logOutputs=off  logFile=C:\Users\ASUS\Desktop\sift_fpga\Octave_2\tb_test_final_sift\test%5Ffinal%5Fsift_sift%5Foctave1_matching_compare%5Fdescriptor_get%5Fdistance_sub%5FGradOrian3_Multiplexer2.fixedpointlog
  Parallel Adder Subtractor : allblocks_alteradspbuilder2/Parallel Adder Subtractor  number_of_inputs=2  direction=+-  use_pipeline=on  pipeline_display=1  phase_selection=1  use_ena=on  use_aclr=off  allowFloatingPointOverride=on  logOutputs=off  logFile=C:\Users\ASUS\Desktop\sift_fpga\Octave_2\tb_test_final_sift\test%5Ffinal%5Fsift_sift%5Foctave1_matching_compare%5Fdescriptor_get%5Fdistance_sub%5FGradOrian3_Parallel+Adder+Subtractor.fixedpointlog
  Parallel Adder Subtractor1 : allblocks_alteradspbuilder2/Parallel Adder Subtractor  number_of_inputs=2  direction=+-  use_pipeline=on  pipeline_display=1  phase_selection=1  use_ena=on  use_aclr=off  allowFloatingPointOverride=on  logOutputs=off  logFile=C:\Users\ASUS\Desktop\sift_fpga\Octave_2\tb_test_final_sift\test%5Ffinal%5Fsift_sift%5Foctave1_matching_compare%5Fdescriptor_get%5Fdistance_sub%5FGradOrian3_Parallel+Adder+Subtractor1.fixedpointlog
  sub_bin : Outport
  wires:
  Comparator3/1 -> Delay/1
  [bin2] -> Comparator3/2
  [bin1] -> Comparator3/1
  Delay/1 -> Multiplexer2/1
  [clken] -> Delay/2
  [bin2] -> Parallel Adder Subtractor/2
  [bin1] -> Parallel Adder Subtractor1/2
  [bin2] -> Parallel Adder Subtractor1/1
  [clken] -> Parallel Adder Subtractor/3
  Parallel Adder Subtractor/1 -> [bin12]
  Parallel Adder Subtractor1/1 -> [bin21]
  [clken] -> Parallel Adder Subtractor1/3
  [bin1] -> Parallel Adder Subtractor/1
  bin1/1 -> [bin1]
  bin2/1 -> [bin2]
  [bin12] -> Multiplexer2/3
  [bin21] -> Multiplexer2/2
  Multiplexer2/1 -> sub_bin/1
  clken/1 -> [clken]

== system test_final_sift/sift_octave1/matching/compare_descriptor/get_distance/sub_GradOrian4 ==
  bin1 : Inport
  bin2 : Inport  Port=2
  clken : Inport  Port=3
  Comparator3 : allblocks_alteradspbuilder2/Comparator  direction=a > b  pipeline_display=0  allowFloatingPointOverride=on  logOutputs=off  logFile=C:\Users\ASUS\Desktop\sift_fpga\Octave_2\tb_test_final_sift\test%5Ffinal%5Fsift_sift%5Foctave1_matching_compare%5Fdescriptor_get%5Fdistance_sub%5FGradOrian4_Comparator3.fixedpointlog
  Delay : allblocks_alteradspbuilder2/Delay  pipeline=1  pipeline_display=1  ClockPhase=1  use_ena=on  use_sclr=off  allowFloatingPointOverride=on  logOutputs=off  logFile=C:\Users\ASUS\Desktop\sift_fpga\Octave_2\tb_test_final_sift\test%5Ffinal%5Fsift_sift%5Foctave1_matching_compare%5Fdescriptor_get%5Fdistance_sub%5FGradOrian4_Delay.fixedpointlog  use_init=off  reset_value=1
  Multiplexer2 : allblocks_alteradspbuilder2/Multiplexer  numInputs=2  pipeline=0  oneHot=off  pipeline_display=0  use_ena=off  use_aclr=off  allowFloatingPointOverride=on  logOutputs=off  logFile=C:\Users\ASUS\Desktop\sift_fpga\Octave_2\tb_test_final_sift\test%5Ffinal%5Fsift_sift%5Foctave1_matching_compare%5Fdescriptor_get%5Fdistance_sub%5FGradOrian4_Multiplexer2.fixedpointlog
  Parallel Adder Subtractor : allblocks_alteradspbuilder2/Parallel Adder Subtractor  number_of_inputs=2  direction=+-  use_pipeline=on  pipeline_display=1  phase_selection=1  use_ena=on  use_aclr=off  allowFloatingPointOverride=on  logOutputs=off  logFile=C:\Users\ASUS\Desktop\sift_fpga\Octave_2\tb_test_final_sift\test%5Ffinal%5Fsift_sift%5Foctave1_matching_compare%5Fdescriptor_get%5Fdistance_sub%5FGradOrian4_Parallel+Adder+Subtractor.fixedpointlog
  Parallel Adder Subtractor1 : allblocks_alteradspbuilder2/Parallel Adder Subtractor  number_of_inputs=2  direction=+-  use_pipeline=on  pipeline_display=1  phase_selection=1  use_ena=on  use_aclr=off  allowFloatingPointOverride=on  logOutputs=off  logFile=C:\Users\ASUS\Desktop\sift_fpga\Octave_2\tb_test_final_sift\test%5Ffinal%5Fsift_sift%5Foctave1_matching_compare%5Fdescriptor_get%5Fdistance_sub%5FGradOrian4_Parallel+Adder+Subtractor1.fixedpointlog
  sub_bin : Outport
  wires:
  Comparator3/1 -> Delay/1
  [bin2] -> Comparator3/2
  [bin1] -> Comparator3/1
  Delay/1 -> Multiplexer2/1
  [clken] -> Delay/2
  [bin2] -> Parallel Adder Subtractor/2
  [bin1] -> Parallel Adder Subtractor1/2
  [bin2] -> Parallel Adder Subtractor1/1
  [clken] -> Parallel Adder Subtractor/3
  Parallel Adder Subtractor/1 -> [bin12]
  Parallel Adder Subtractor1/1 -> [bin21]
  [clken] -> Parallel Adder Subtractor1/3
  [bin1] -> Parallel Adder Subtractor/1
  bin1/1 -> [bin1]
  bin2/1 -> [bin2]
  [bin12] -> Multiplexer2/3
  [bin21] -> Multiplexer2/2
  Multiplexer2/1 -> sub_bin/1
  clken/1 -> [clken]

== system test_final_sift/sift_octave1/matching/compare_descriptor/get_distance/sub_GradOrian5 ==
  bin1 : Inport
  bin2 : Inport  Port=2
  clken : Inport  Port=3
  Comparator3 : allblocks_alteradspbuilder2/Comparator  direction=a > b  pipeline_display=0  allowFloatingPointOverride=on  logOutputs=off  logFile=C:\Users\ASUS\Desktop\sift_fpga\Octave_2\tb_test_final_sift\test%5Ffinal%5Fsift_sift%5Foctave1_matching_compare%5Fdescriptor_get%5Fdistance_sub%5FGradOrian5_Comparator3.fixedpointlog
  Delay : allblocks_alteradspbuilder2/Delay  pipeline=1  pipeline_display=1  ClockPhase=1  use_ena=on  use_sclr=off  allowFloatingPointOverride=on  logOutputs=off  logFile=C:\Users\ASUS\Desktop\sift_fpga\Octave_2\tb_test_final_sift\test%5Ffinal%5Fsift_sift%5Foctave1_matching_compare%5Fdescriptor_get%5Fdistance_sub%5FGradOrian5_Delay.fixedpointlog  use_init=off  reset_value=1
  Multiplexer2 : allblocks_alteradspbuilder2/Multiplexer  numInputs=2  pipeline=0  oneHot=off  pipeline_display=0  use_ena=off  use_aclr=off  allowFloatingPointOverride=on  logOutputs=off  logFile=C:\Users\ASUS\Desktop\sift_fpga\Octave_2\tb_test_final_sift\test%5Ffinal%5Fsift_sift%5Foctave1_matching_compare%5Fdescriptor_get%5Fdistance_sub%5FGradOrian5_Multiplexer2.fixedpointlog
  Parallel Adder Subtractor : allblocks_alteradspbuilder2/Parallel Adder Subtractor  number_of_inputs=2  direction=+-  use_pipeline=on  pipeline_display=1  phase_selection=1  use_ena=on  use_aclr=off  allowFloatingPointOverride=on  logOutputs=off  logFile=C:\Users\ASUS\Desktop\sift_fpga\Octave_2\tb_test_final_sift\test%5Ffinal%5Fsift_sift%5Foctave1_matching_compare%5Fdescriptor_get%5Fdistance_sub%5FGradOrian5_Parallel+Adder+Subtractor.fixedpointlog
  Parallel Adder Subtractor1 : allblocks_alteradspbuilder2/Parallel Adder Subtractor  number_of_inputs=2  direction=+-  use_pipeline=on  pipeline_display=1  phase_selection=1  use_ena=on  use_aclr=off  allowFloatingPointOverride=on  logOutputs=off  logFile=C:\Users\ASUS\Desktop\sift_fpga\Octave_2\tb_test_final_sift\test%5Ffinal%5Fsift_sift%5Foctave1_matching_compare%5Fdescriptor_get%5Fdistance_sub%5FGradOrian5_Parallel+Adder+Subtractor1.fixedpointlog
  sub_bin : Outport
  wires:
  Comparator3/1 -> Delay/1
  [bin2] -> Comparator3/2
  [bin1] -> Comparator3/1
  Delay/1 -> Multiplexer2/1
  [clken] -> Delay/2
  [bin2] -> Parallel Adder Subtractor/2
  [bin1] -> Parallel Adder Subtractor1/2
  [bin2] -> Parallel Adder Subtractor1/1
  [clken] -> Parallel Adder Subtractor/3
  Parallel Adder Subtractor/1 -> [bin12]
  Parallel Adder Subtractor1/1 -> [bin21]
  [clken] -> Parallel Adder Subtractor1/3
  [bin1] -> Parallel Adder Subtractor/1
  bin1/1 -> [bin1]
  bin2/1 -> [bin2]
  [bin12] -> Multiplexer2/3
  [bin21] -> Multiplexer2/2
  Multiplexer2/1 -> sub_bin/1
  clken/1 -> [clken]

== system test_final_sift/sift_octave1/matching/compare_descriptor/get_distance/sub_GradOrian6 ==
  bin1 : Inport
  bin2 : Inport  Port=2
  clken : Inport  Port=3
  Comparator3 : allblocks_alteradspbuilder2/Comparator  direction=a > b  pipeline_display=0  allowFloatingPointOverride=on  logOutputs=off  logFile=C:\Users\ASUS\Desktop\sift_fpga\Octave_2\tb_test_final_sift\test%5Ffinal%5Fsift_sift%5Foctave1_matching_compare%5Fdescriptor_get%5Fdistance_sub%5FGradOrian6_Comparator3.fixedpointlog
  Delay : allblocks_alteradspbuilder2/Delay  pipeline=1  pipeline_display=1  ClockPhase=1  use_ena=on  use_sclr=off  allowFloatingPointOverride=on  logOutputs=off  logFile=C:\Users\ASUS\Desktop\sift_fpga\Octave_2\tb_test_final_sift\test%5Ffinal%5Fsift_sift%5Foctave1_matching_compare%5Fdescriptor_get%5Fdistance_sub%5FGradOrian6_Delay.fixedpointlog  use_init=off  reset_value=1
  Multiplexer2 : allblocks_alteradspbuilder2/Multiplexer  numInputs=2  pipeline=0  oneHot=off  pipeline_display=0  use_ena=off  use_aclr=off  allowFloatingPointOverride=on  logOutputs=off  logFile=C:\Users\ASUS\Desktop\sift_fpga\Octave_2\tb_test_final_sift\test%5Ffinal%5Fsift_sift%5Foctave1_matching_compare%5Fdescriptor_get%5Fdistance_sub%5FGradOrian6_Multiplexer2.fixedpointlog
  Parallel Adder Subtractor : allblocks_alteradspbuilder2/Parallel Adder Subtractor  number_of_inputs=2  direction=+-  use_pipeline=on  pipeline_display=1  phase_selection=1  use_ena=on  use_aclr=off  allowFloatingPointOverride=on  logOutputs=off  logFile=C:\Users\ASUS\Desktop\sift_fpga\Octave_2\tb_test_final_sift\test%5Ffinal%5Fsift_sift%5Foctave1_matching_compare%5Fdescriptor_get%5Fdistance_sub%5FGradOrian6_Parallel+Adder+Subtractor.fixedpointlog
  Parallel Adder Subtractor1 : allblocks_alteradspbuilder2/Parallel Adder Subtractor  number_of_inputs=2  direction=+-  use_pipeline=on  pipeline_display=1  phase_selection=1  use_ena=on  use_aclr=off  allowFloatingPointOverride=on  logOutputs=off  logFile=C:\Users\ASUS\Desktop\sift_fpga\Octave_2\tb_test_final_sift\test%5Ffinal%5Fsift_sift%5Foctave1_matching_compare%5Fdescriptor_get%5Fdistance_sub%5FGradOrian6_Parallel+Adder+Subtractor1.fixedpointlog
  sub_bin : Outport
  wires:
  Comparator3/1 -> Delay/1
  [bin2] -> Comparator3/2
  [bin1] -> Comparator3/1
  Delay/1 -> Multiplexer2/1
  [clken] -> Delay/2
  [bin2] -> Parallel Adder Subtractor/2
  [bin1] -> Parallel Adder Subtractor1/2
  [bin2] -> Parallel Adder Subtractor1/1
  [clken] -> Parallel Adder Subtractor/3
  Parallel Adder Subtractor/1 -> [bin12]
  Parallel Adder Subtractor1/1 -> [bin21]
  [clken] -> Parallel Adder Subtractor1/3
  [bin1] -> Parallel Adder Subtractor/1
  bin1/1 -> [bin1]
  bin2/1 -> [bin2]
  [bin12] -> Multiplexer2/3
  [bin21] -> Multiplexer2/2
  Multiplexer2/1 -> sub_bin/1
  clken/1 -> [clken]
